simulink model "ejercicio6_09_02_17"  (R2013a)
settings: Solver=FixedStepDiscrete  StartTime=0.0  StopTime=139  RelTol=1e-3
settings Model: Creator=Miguel  LastModifiedBy=Miguel

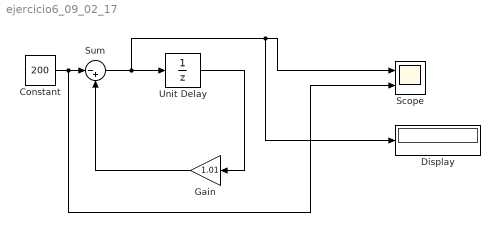
== system ejercicio6_09_02_17 ==
  Constant : Constant  Value=200
  Display : Display
  Gain : Gain  Gain=1.01  SampleTime=1
  Scope : Scope  NumInputPorts=2
      settings: YMin=-5~-5  YMax=5~5
  Sum : Sum  Inputs=|-+
  Unit Delay : UnitDelay  InitialCondition=15000
  wires:
  Sum/1 -> Display/1, Scope/1, Unit Delay/1
  Gain/1 -> Sum/2
  Unit Delay/1 -> Gain/1
  Constant/1 -> Scope/2, Sum/1
